simulink model "hover_prop_table"  (R2025b)
settings: Solver=VariableStepAuto  StartTime=0.0  StopTime=10.0  RelTol=1e-3
PreLoadFcn:
  | d=fileparts(get_param(bdroot,'FileName')); addpath(d); hover_2d_to_workspace;
InitFcn:
  | d=fileparts(get_param(bdroot,'FileName')); addpath(d); hover_2d_to_workspace;
undefined symbols (not defined in the file or in its folder): cfd2d_D, cfd2d_ja, cfd2d_jl, cfd2d_kQ, cfd2d_kT, cfd2d_P1_CEF_X, cfd2d_P1_CEF_Y, cfd2d_P1_CEF_Z, cfd2d_P1_CEM_X, cfd2d_P1_CEM_Y, cfd2d_P1_CEM_Z, cfd2d_P5_CEF_X, cfd2d_P5_CEF_Y, cfd2d_P5_CEF_Z, cfd2d_P5_CEM_X, cfd2d_P5_CEM_Y, cfd2d_P5_CEM_Z, cfd2d_rho, cfd3d_aInf, cfd3d_D
libraries: sharedtransform x2
settings Model: Creator=someone  LastModifiedBy=someone

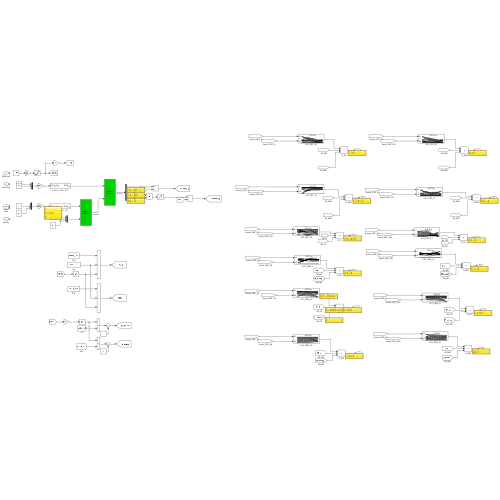
[thumbnail: Simulink's stored preview of the top-level diagram]
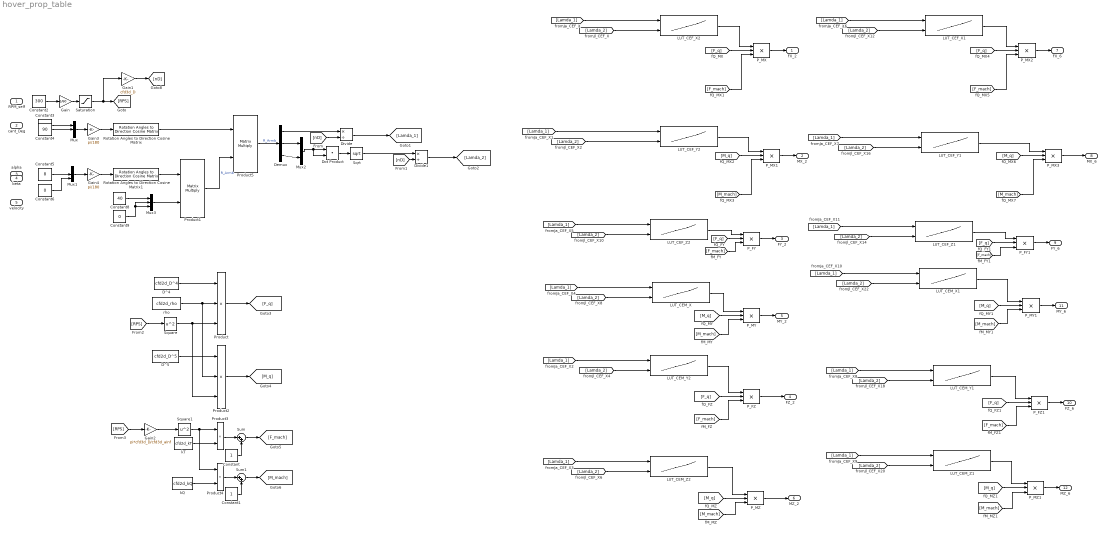
== system hover_prop_table ==
  RPM_self : Inport
  cant_Deg : Inport  Port=2
  alpha : Inport  Port=3
  beta : Inport  Port=4
  velocity : Inport  Port=5
  Constant : Constant
  Constant1 : Constant
  Constant2 : Constant  Value=300
  Constant3 : Constant  Value=7
  Constant4 : Constant  Value=90
  Constant5 : Constant  Value=8
  Constant6 : Constant  Value=0
  Constant8 : Constant  Value=40
  Constant9 : Constant  Value=0
  D^4 : Constant  Value=cfd2d_D^4
  D^5 : Constant  Value=cfd2d_D^5
  Demux : Demux  Outputs=3
  Divide : Product  Inputs=*/
  Divide1 : Product  Inputs=*/
  Dot Product : DotProduct  OutDataTypeStr=Inherit: Inherit via internal rule
  Gain : Gain  Gain=1/60
  Gain1 : Gain  Gain=cfd3d_D
  Gain2 : Gain  Gain=pi*cfd3d_D/cfd3d_aInf
  Gain3 : Gain  Gain=pi/180
  Gain4 : Gain  Gain=pi/180
  LUT_CEF_X1 : Lookup_n-D  BreakpointsForDimension1=cfd2d_ja  BreakpointsForDimension2=cfd2d_jl  BreakpointsForDimension3=[5, 7]  Table=cfd2d_P5_CEF_X  ExtrapMethod=Clip  UseLastTableValue=on  InternalRulePriority=Speed  RndMeth=Simplest
      settings: InputPortMap=u0,u1
  LUT_CEF_X2 : Lookup_n-D  BreakpointsForDimension1=cfd2d_ja  BreakpointsForDimension2=cfd2d_jl  BreakpointsForDimension3=[5, 7]  Table=cfd2d_P1_CEF_X  ExtrapMethod=Clip  UseLastTableValue=on  InternalRulePriority=Speed  RndMeth=Simplest
      settings: InputPortMap=u0,u1
  LUT_CEF_Y1 : Lookup_n-D  BreakpointsForDimension1=cfd2d_ja  BreakpointsForDimension2=cfd2d_jl  BreakpointsForDimension3=[5, 7]  Table=cfd2d_P5_CEM_X  ExtrapMethod=Clip  UseLastTableValue=on  InternalRulePriority=Speed  RndMeth=Simplest
      settings: InputPortMap=u0,u1
  LUT_CEF_Y2 : Lookup_n-D  BreakpointsForDimension1=cfd2d_ja  BreakpointsForDimension2=cfd2d_jl  BreakpointsForDimension3=[5, 7]  Table=cfd2d_P1_CEM_X  ExtrapMethod=Clip  UseLastTableValue=on  InternalRulePriority=Speed  RndMeth=Simplest
      settings: InputPortMap=u0,u1
  LUT_CEF_Z1 : Lookup_n-D  BreakpointsForDimension1=cfd2d_ja  BreakpointsForDimension2=cfd2d_jl  BreakpointsForDimension3=[5, 7]  Table=cfd2d_P5_CEF_Y  ExtrapMethod=Clip  UseLastTableValue=on  InternalRulePriority=Speed  RndMeth=Simplest
      settings: InputPortMap=u0,u1
  LUT_CEF_Z2 : Lookup_n-D  BreakpointsForDimension1=cfd2d_ja  BreakpointsForDimension2=cfd2d_jl  BreakpointsForDimension3=[5, 7]  Table=cfd2d_P1_CEF_Y  ExtrapMethod=Clip  UseLastTableValue=on  InternalRulePriority=Speed  RndMeth=Simplest
      settings: InputPortMap=u0,u1
  LUT_CEM_X : Lookup_n-D  BreakpointsForDimension1=cfd2d_ja  BreakpointsForDimension2=cfd2d_jl  BreakpointsForDimension3=[5, 7]  Table=cfd2d_P1_CEM_Y  ExtrapMethod=Clip  UseLastTableValue=on  InternalRulePriority=Speed  RndMeth=Simplest
      settings: InputPortMap=u0,u1
  LUT_CEM_X1 : Lookup_n-D  BreakpointsForDimension1=cfd2d_ja  BreakpointsForDimension2=cfd2d_jl  BreakpointsForDimension3=[5, 7]  Table=cfd2d_P5_CEM_Y  ExtrapMethod=Clip  UseLastTableValue=on  InternalRulePriority=Speed  RndMeth=Simplest
      settings: InputPortMap=u0,u1
  LUT_CEM_Y1 : Lookup_n-D  BreakpointsForDimension1=cfd2d_ja  BreakpointsForDimension2=cfd2d_jl  BreakpointsForDimension3=[5, 7]  Table=cfd2d_P5_CEF_Z  ExtrapMethod=Clip  UseLastTableValue=on  InternalRulePriority=Speed  RndMeth=Simplest
      settings: InputPortMap=u0,u1
  LUT_CEM_Y2 : Lookup_n-D  BreakpointsForDimension1=cfd2d_ja  BreakpointsForDimension2=cfd2d_jl  BreakpointsForDimension3=[5, 7]  Table=cfd2d_P1_CEF_Z  ExtrapMethod=Clip  UseLastTableValue=on  InternalRulePriority=Speed  RndMeth=Simplest
      settings: InputPortMap=u0,u1
  LUT_CEM_Z1 : Lookup_n-D  BreakpointsForDimension1=cfd2d_ja  BreakpointsForDimension2=cfd2d_jl  BreakpointsForDimension3=[5, 7]  Table=cfd2d_P5_CEM_Z  ExtrapMethod=Clip  UseLastTableValue=on  InternalRulePriority=Speed  RndMeth=Simplest
      settings: InputPortMap=u0,u1
  LUT_CEM_Z2 : Lookup_n-D  BreakpointsForDimension1=cfd2d_ja  BreakpointsForDimension2=cfd2d_jl  BreakpointsForDimension3=[5, 7]  Table=cfd2d_P1_CEM_Z  ExtrapMethod=Clip  UseLastTableValue=on  InternalRulePriority=Speed  RndMeth=Simplest
      settings: InputPortMap=u0,u1
  Mux : Mux  Inputs=3
  Mux1 : Mux  Inputs=3
  Mux2 : Mux  Inputs=2
  Mux3 : Mux  Inputs=3
  P_FY : Product  Inputs=***
  P_FY1 : Product  Inputs=***
  P_FZ : Product  Inputs=***
  P_FZ1 : Product  Inputs=***
  P_MX{,1..3} (4 alike) : Product  Inputs=***
  P_MY : Product  Inputs=***
  P_MY1 : Product  Inputs=***
  P_MZ : Product  Inputs=***
  P_MZ1 : Product  Inputs=***
  Product : Product  Inputs=3
  Product1 : Product  Multiplication=Matrix(*)  InputSameDT=on  SaturateOnIntegerOverflow=on  OutDataTypeStr=Inherit: Same as first input
  Product2 : Product  Inputs=3
  Product3 : Product
  Product4 : Product
  Product5 : Product  Multiplication=Matrix(*)  InputSameDT=on  SaturateOnIntegerOverflow=on  OutDataTypeStr=Inherit: Same as first input
  Rotation Angles to Direction Cosine Matrix : sharedtransform/Rotation Angles to Direction Cosine Matrix  rotationOrder=ZYX  aMode=aMode
  Rotation Angles to Direction Cosine Matrix1 : sharedtransform/Rotation Angles to Direction Cosine Matrix  rotationOrder=ZYX  aMode=aMode
  Saturation : Saturate  UpperLimit=inf  LowerLimit=1e-4
  Sqrt : Sqrt
  Square : Math  Operator=square
  Square1 : Math  Operator=square
  Sum : Sum  Inputs=|++
  Sum1 : Sum  Inputs=|++
  kQ : Constant  Value=cfd2d_kQ
  kT : Constant  Value=cfd2d_kT
  rho : Constant  Value=cfd2d_rho
  FX_2 : Outport
  MX_2 : Outport  Port=2
  FY_2 : Outport  Port=3
  FZ_2 : Outport  Port=4
  MY_2 : Outport  Port=5
  MZ_2 : Outport  Port=6
  FX_6 : Outport  Port=7
  MX_6 : Outport  Port=8
  FY_6 : Outport  Port=9
  FZ_6 : Outport  Port=10
  MY_6 : Outport  Port=11
  MZ_6 : Outport  Port=12
  wires:
  Constant6/1 -> Mux1/3
  Constant5/1 -> Mux1/2
  Gain3/1 -> Rotation Angles to Direction Cosine Matrix/1
  Constant8/1 -> Mux3/1
  Gain4/1 -> Rotation Angles to Direction Cosine Matrix1/1
  [Lamda_2] -> LUT_CEM_Z2/2
  [Lamda_1] -> LUT_CEM_Z2/1
  [F_mach] -> P_MX/3
  Sum/1 -> [F_mach]
  Constant1/1 -> Sum1/2
  Product5/1 -> Demux/1  "R_Armb"
  [F_q] -> P_FZ/2
  [F_mach] -> P_FZ/3
  P_FY/1 -> FY_2/1
  LUT_CEF_Z2/1 -> P_FY/1
  LUT_CEM_X/1 -> P_MY/1
  [M_q] -> P_MZ/2
  [F_q] -> P_FY/2
  LUT_CEM_Y2/1 -> P_FZ/1
  LUT_CEM_Z2/1 -> P_MZ/1
  [M_mach] -> P_MY/3
  P_MZ/1 -> MZ_2/1
  Constant9/1 -> Mux3/3, Mux3/2
  [RPS] -> Gain2/1
  [Lamda_1] -> LUT_CEM_X/1
  [Lamda_2] -> LUT_CEM_X/2
  Constant2/1 -> Gain/1
  [Lamda_1] -> LUT_CEF_Z2/1
  Gain2/1 -> Square1/1
  Gain1/1 -> [nD]
  Mux3/1 -> Product1/2
  [F_q] -> P_FZ1/2
  [M_q] -> P_MZ1/2
  P_MX2/1 -> FX_6/1
  LUT_CEF_Y1/1 -> P_MX3/1
  [M_q] -> P_MX3/2
  P_FZ1/1 -> FZ_6/1
  [Lamda_2] -> LUT_CEM_Y1/2
  [Lamda_1] -> LUT_CEF_Y1/1
  [Lamda_1] -> LUT_CEF_Z1/1
  [F_q] -> P_MX2/2
  [Lamda_1] -> LUT_CEF_X1/1
  [Lamda_2] -> LUT_CEF_X1/2
  [M_mach] -> P_MX3/3
  P_MX3/1 -> MX_6/1
  LUT_CEF_X1/1 -> P_MX2/1
  [Lamda_1] -> LUT_CEM_Y1/1
  [Lamda_2] -> LUT_CEF_Z1/2
  [Lamda_2] -> LUT_CEM_X1/2
  [F_mach] -> P_FY1/3
  LUT_CEF_Z1/1 -> P_FY1/1
  P_MZ1/1 -> MZ_6/1
  [F_mach] -> P_FY/3
  LUT_CEM_Z1/1 -> P_MZ1/1
  P_MY1/1 -> MY_6/1
  [F_q] -> P_FY1/2
  LUT_CEM_X1/1 -> P_MY1/1
  [M_mach] -> P_MZ/3
  [M_mach] -> P_MY1/3
  LUT_CEM_Y1/1 -> P_FZ1/1
  [F_mach] -> P_FZ1/3
  [F_mach] -> P_MX2/3
  [nD] -> Divide/2
  [Lamda_2] -> LUT_CEF_Z2/2
  D^4/1 -> Product/1
  Mux1/1 -> Gain4/1
  [Lamda_1] -> LUT_CEM_Y2/1
  Product2/1 -> [M_q]
  Mux/1 -> Gain3/1
  [Lamda_2] -> LUT_CEF_X2/2
  Demux/3 -> Mux2/2
  LUT_CEF_X2/1 -> P_MX/1
  Product/1 -> [F_q]
  kQ/1 -> Product4/2
  [M_mach] -> P_MZ1/3
  Demux/1 -> Divide/1
  kT/1 -> Product3/2
  Demux/2 -> Mux2/1
  [Lamda_1] -> LUT_CEM_Z1/1
  P_MX1/1 -> MX_2/1
  [M_mach] -> P_MX1/3
  LUT_CEF_Y2/1 -> P_MX1/1
  P_FZ/1 -> FZ_2/1
  [M_q] -> P_MX1/2
  [Lamda_2] -> LUT_CEF_Y2/2
  Product4/1 -> Sum1/1
  D^5/1 -> Product2/1
  [Lamda_1] -> LUT_CEF_Y2/1
  [Lamda_2] -> LUT_CEM_Z1/2
  Rotation Angles to Direction Cosine Matrix/1 -> Product5/1
  Constant/1 -> Sum/2
  [nD] -> Divide1/2
  [Lamda_1] -> LUT_CEF_X2/1
  Rotation Angles to Direction Cosine Matrix1/1 -> Product1/1
  Mux2/1 -> Dot Product/2, Dot Product/1
  rho/1 -> Product2/2, Product/2
  Square1/1 -> Product4/1, Product3/1
  [RPS] -> Square/1
  [M_q] -> P_MY/2
  Sum1/1 -> [M_mach]
  Product3/1 -> Sum/1
  [Lamda_1] -> LUT_CEM_X1/1
  P_MY/1 -> MY_2/1
  Gain/1 -> Saturation/1
  Square/1 -> Product2/3, Product/3
  Dot Product/1 -> Sqrt/1
  P_FY1/1 -> FY_6/1
  Constant3/1 -> Mux/1
  Product1/1 -> Product5/2  "R_Armb"
  Divide1/1 -> [Lamda_2]
  Divide/1 -> [Lamda_1]
  Sqrt/1 -> Divide1/1
  [M_q] -> P_MY1/2
  [F_q] -> P_MX/2
  [Lamda_2] -> LUT_CEF_Y1/2
  P_MX/1 -> FX_2/1
  [Lamda_2] -> LUT_CEM_Y2/2
  Constant4/1 -> Mux/2
  Saturation/1 -> Gain1/1, [RPS]
